simulink model "Example_2_Disturbance_Estimation_Mdl"  (Simulink 7.1)
settings: Solver=ode23s  StartTime=0.0  StopTime=5  RelTol=1e-3
values from neighbouring files (symbols this model uses):
  A = sys.a    [Example_2_Control.m]    (also in Example_2_Discretization.m; Example_2_Disturbance_Estimation.m; Example_2_Integral_Control.m; Example_2_Prediction_Observer.m)
  a = 0.1    [Example_2_Disturbance_Estimation.m]
  A_aug = [A B_w*C_w; zeros(n_w,n) A_w]    [Example_2_Disturbance_Estimation.m]    (also in Example_2_Integral_Control.m = [1 C; zeros(n,1) A])
  B = sys.b    [Example_2_Control.m]    (also in Example_2_Discretization.m; Example_2_Disturbance_Estimation.m; Example_2_Integral_Control.m; Example_2_Prediction_Observer.m)
  B_aug = [B; zeros(n_w,m)]    [Example_2_Disturbance_Estimation.m]    (also in Example_2_Integral_Control.m = [0; B])
  B_w = sys_d.b    [Example_2_Control.m]    (also in Example_2_Discretization.m; Example_2_Disturbance_Estimation.m; Example_2_Integral_Control.m; Example_2_Prediction_Observer.m)
  B_w_aug = [B_w; zeros(n_w,m)]    [Example_2_Disturbance_Estimation.m]
  C = sys.c    [Example_2_Control.m]    (also in Example_2_Discretization.m; Example_2_Disturbance_Estimation.m; Example_2_Integral_Control.m; Example_2_Prediction_Observer.m)
  C_aug = [C zeros(p,n_w)]    [Example_2_Disturbance_Estimation.m]
  D = sys.d    [Example_2_Control.m]    (also in Example_2_Discretization.m; Example_2_Disturbance_Estimation.m; Example_2_Integral_Control.m; Example_2_Prediction_Observer.m)
  D_aug = D    [Example_2_Disturbance_Estimation.m]
  h = T_r/N_r    [Example_2_Control.m]    (also in Example_2_Discretization.m; Example_2_Disturbance_Estimation.m; Example_2_Integral_Control.m; Example_2_Prediction_Observer.m)
  K = -K    [Example_2_Control.m]    (also in Example_2_Disturbance_Estimation.m; Example_2_Integral_Control.m = -K_aug(2:n_aug); Example_2_Reference_Tracking.m; Example_4_Active_Suspension_System.m)
  L = L'    [Example_2_Disturbance_Estimation.m]    (also in Example_2_Prediction_Observer.m)
  omega = 2*pi/T    (= 13.962634016)    [Example_2_Disturbance_Estimation.m]
  T = l/v    (= 0.45)    [Example_2_Disturbance_Estimation.m]
  x_0 = [0; 0; 0; 0]    [Example_2_Analysis.m]    (also in Example_2_Control.m = [25*9.81/k_s; 0; 25*9.81/k_u; 0]; Example_2_Discretization.m = [25*9.81/k_s; 0; 25*9.81/k_u; 0]; Example_2_Disturbance_Estimation.m; Example_2_Integral_Control.m)
  x_0_obsv = [0; 0; 0; 0; 0; 0]    [Example_2_Disturbance_Estimation.m]    (also in Example_2_Prediction_Observer.m = [0; 0; 0; 0])
settings Model: Creator=d_goerges  LastModifiedBy=d_goerges
settings DataIOCC: Refine=10
settings OptimizationCC: InitFltsAndDblsToZero=off
settings DebuggingCC: FcnCallInpInsideContextMsg=Enable All  StrictBusMsg=ErrorLevel1
settings GRTTargetCC: CPPClassGenCompliant=off

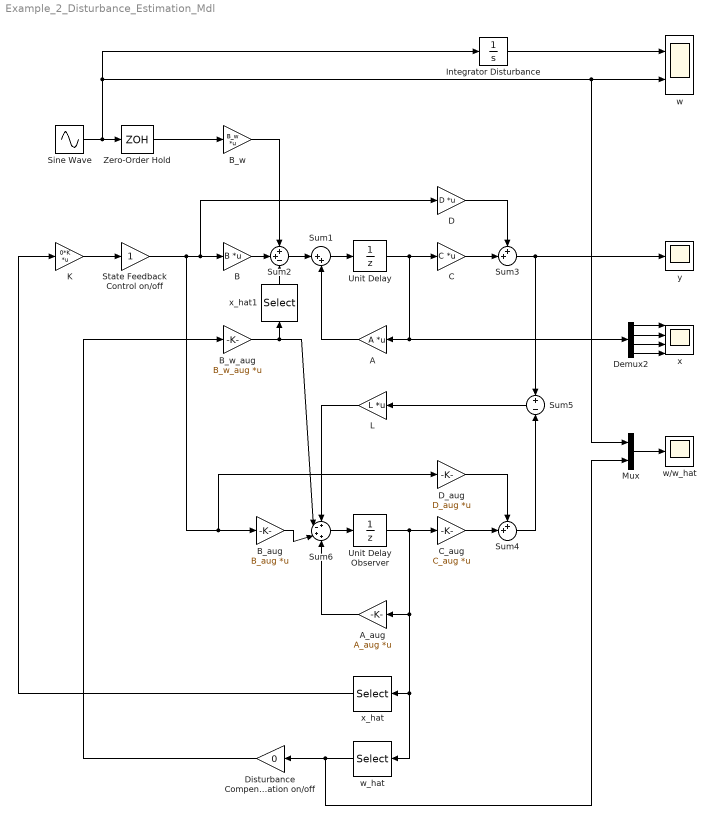
== system Example_2_Disturbance_Estimation_Mdl ==
  A : Gain  Orientation=left  Gain=A  Multiplication=Matrix(K*u)
  A_aug : Gain  Orientation=left  Gain=A_aug  Multiplication=Matrix(K*u)
  B : Gain  Gain=B  Multiplication=Matrix(K*u)
  B_aug : Gain  Gain=B_aug  Multiplication=Matrix(K*u)
  B_w : Gain  Gain=B_w  Multiplication=Matrix(K*u)  SampleTime=h
  B_w_aug : Gain  Gain=B_w_aug  Multiplication=Matrix(K*u)  SampleTime=h
  C : Gain  Gain=C  Multiplication=Matrix(K*u)
  C_aug : Gain  Gain=C_aug  Multiplication=Matrix(K*u)
  D : Gain  Gain=D  Multiplication=Matrix(K*u)
  D_aug : Gain  Gain=D_aug  Multiplication=Matrix(K*u)
  Demux2 : Demux
  Disturbance Compensation on/off : Gain  Orientation=left  Gain=0
  Integrator Disturbance : Integrator
  K : Gain  Gain=0*K  Multiplication=Matrix(K*u)
  L : Gain  Orientation=left  Gain=L  Multiplication=Matrix(K*u)
  Mux : Mux  Inputs=2
  Sine Wave : Sin  Amplitude=a*2*pi/T  Frequency=omega  Phase=pi/2  SampleTime=0
  State Feedback Control on/off : Gain
  Sum1 : Sum  Inputs=|++
  Sum2 : Sum  Inputs=++-
  Sum3 : Sum  Inputs=++|
  Sum4 : Sum  Inputs=++|
  Sum5 : Sum  Orientation=left  Inputs=+|-
  Sum6 : Sum  Inputs=+-++
  Unit Delay : UnitDelay  X0=x_0  SampleTime=h
  Unit Delay Observer : UnitDelay  X0=x_0_obsv  SampleTime=h
  Zero-Order Hold : ZeroOrderHold  SampleTime=h
  w : Scope  NumInputPorts=2
      settings: YMin=-5~-5  YMax=5~5  SaveName=ScopeData2
  w/w_hat : Scope
      settings: SaveName=ScopeData4
  w_hat : Selector  Orientation=left  InputPortWidth=6  IndexOptions=Index vector (dialog)  Indices=5  OutputSizes=1
  x : Scope  NumInputPorts=4
      settings: YMin=-5~-5~-5~-5  YMax=5~5~5~5
  x_hat : Selector  Orientation=left  InputPortWidth=6  IndexOptions=Index vector (dialog)  Indices=1:4  OutputSizes=1
  x_hat1 : Selector  Orientation=up  InputPortWidth=6  IndexOptions=Index vector (dialog)  Indices=1:4  OutputSizes=1
  y : Scope
  wires:
  C/1 -> Sum3/2
  Sum3/1 -> Sum5/1, y/1
  Unit Delay/1 -> C/1, A/1, Demux2/1
  Sum6/1 -> Unit Delay Observer/1
  C_aug/1 -> Sum4/2
  Unit Delay Observer/1 -> C_aug/1, A_aug/1, x_hat/1, w_hat/1
  K/1 -> State Feedback Control on/off/1
  Sum4/1 -> Sum5/2
  L/1 -> Sum6/1
  Sum5/1 -> L/1
  B_w/1 -> Sum2/1
  Zero-Order Hold/1 -> B_w/1
  Sine Wave/1 -> Zero-Order Hold/1, Integrator Disturbance/1, w/2, Mux/1
  Mux/1 -> w/w_hat/1
  D/1 -> Sum3/1
  D_aug/1 -> Sum4/1
  Integrator Disturbance/1 -> w/1
  w_hat/1 -> Mux/2, Disturbance Compensation on/off/1
  B/1 -> Sum2/2
  Demux2/1 -> x/1
  Demux2/2 -> x/2
  Demux2/3 -> x/3
  Demux2/4 -> x/4
  Sum1/1 -> Unit Delay/1
  A/1 -> Sum1/2
  Sum2/1 -> Sum1/1
  A_aug/1 -> Sum6/4
  B_aug/1 -> Sum6/3
  B_w_aug/1 -> Sum6/2, x_hat1/1
  x_hat1/1 -> Sum2/3
  x_hat/1 -> K/1
  Disturbance Compensation on/off/1 -> B_w_aug/1
  State Feedback Control on/off/1 -> B_aug/1, D_aug/1, B/1, D/1
